simulink model "data_acquisition_file_slider"  (R2019b)
settings: Solver=VariableStepAuto  StartTime=0.0  StopTime=inf  RelTol=1e-3
settings Model: EnablePacing=on  Creator=mandl  LastModifiedBy=mandl

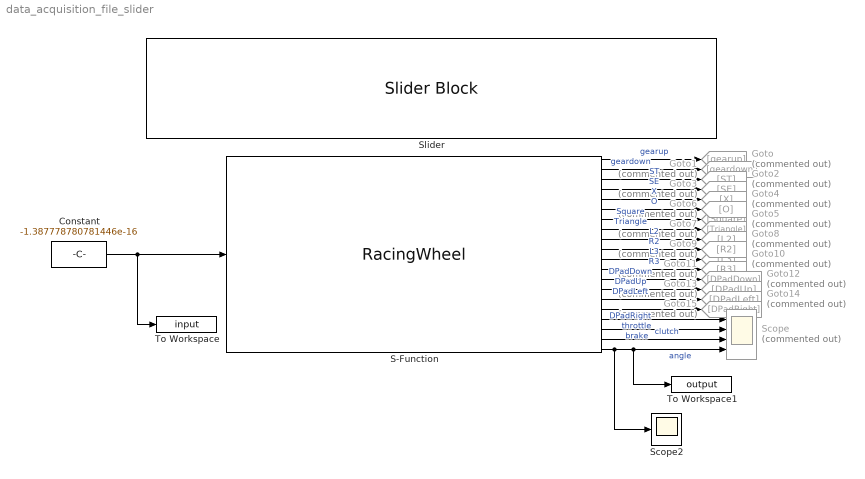
== system data_acquisition_file_slider ==
  Constant : Constant  Value=-1.387778780781446e-16
  Goto : Goto  Commented=on  GotoTag=gearup
  Goto1 : Goto  Commented=on  GotoTag=geardown
  Goto10 : Goto  Commented=on  GotoTag=L3
  Goto11 : Goto  Commented=on  GotoTag=R3
  Goto12 : Goto  Commented=on  GotoTag=DPadDown
  Goto13 : Goto  Commented=on  GotoTag=DPadUp
  Goto14 : Goto  Commented=on  GotoTag=DPadLeft
  Goto15 : Goto  Commented=on  GotoTag=DPadRight
  Goto2 : Goto  Commented=on  GotoTag=ST
  Goto3 : Goto  Commented=on  GotoTag=SE
  Goto4 : Goto  Commented=on  GotoTag=X
  Goto5 : Goto  Commented=on  GotoTag=Square
  Goto6 : Goto  Commented=on  GotoTag=O
  Goto7 : Goto  Commented=on  GotoTag=Triangle
  Goto8 : Goto  Commented=on  GotoTag=L2
  Goto9 : Goto  Commented=on  GotoTag=R2
  S-Function : S-Function  FunctionName=RacingWheel  Parameters=Ts_FF  SFunctionModules=RacingWheel_wrapper  SFunctionDeploymentMode=off  EnableBusSupport=off  mask(Racing Wheel with Force Feedback){Ts_FF=0.01}
      mask prompts: Ts_FF "Constant Force-Feedback Sample Time"
      mask help: Interacts with the windows gaming API from UWP. The force feedback effect is constant over the user defined sampling time below.
      mask init:
      | val = [[.9  0.75 0.75 1 1 .9 .9 1]',[1 1 0.75 0.75 .9 .9 1 .9]'];try , sys = get_param(gcb,'SfunBuilderFcnName');if isempty(sys), sys = get_param(gcb,'FunctionName'); end,catch, sys = get_param(gcb,'FunctionName'); end
      mask Display:
      | plot(val(:,1),val(:,2)),disp(sys),
      | image('icon.png'),
      | port_label('input',1,'FF'),
      | port_label('output',1,'gearup'),
      | port_label('output',2,'geardown'),
      | port_label('output',3,'ST'),
      | port_label('output',4,'SE'),
      | port_label('output',5,'X'),
      | port_label('output',6,'O'),
      | port_label('output',7,'Square'),
      | port_label('output',8,'Triangle'),
      | port_label('output',9,'L2'),
      | port_label('output',10,'R2'),
      | port_label('output',11,'L3'),
      | port_label('output',12,'R3'),
      | port_label('output',13,'DPadDown'),
      | port_label('output',14,'DPadUp'),
      | port_label('output',15,'DPadLeft'),
      | port_label('output',16,'DPadRight'),
      | port_label('output',17,'throttle'),
      | port_label('output',18,'brake'),
      | port_label('output',19,'clutch'),
      | port_label('output',20,'angle')
  Scope : Scope  Commented=on  NumInputPorts=4
  Scope2 : Scope
  Slider : SliderBlock  ScaleMin=-1  ScaleMax=1  TickInterval=0.1
  To Workspace : ToWorkspace  VariableName=input  SaveFormat=Structure With Time  SampleTime=0.01
  To Workspace1 : ToWorkspace  VariableName=output  SaveFormat=Structure With Time  SampleTime=0.01
  wires:
  S-Function/20 -> Scope2/1, To Workspace1/1, Scope/4  "angle"
  S-Function/19 -> Scope/3  "clutch"
  S-Function/18 -> Scope/2  "brake"
  S-Function/17 -> Scope/1  "throttle"
  S-Function/1 -> Goto/1  "gearup"
  S-Function/2 -> Goto1/1  "geardown"
  S-Function/3 -> Goto2/1  "ST"
  S-Function/4 -> Goto3/1  "SE"
  S-Function/5 -> Goto4/1  "X"
  S-Function/6 -> Goto6/1  "O"
  S-Function/7 -> Goto5/1  "Square"
  S-Function/8 -> Goto7/1  "Triangle"
  S-Function/9 -> Goto8/1  "L2"
  S-Function/10 -> Goto9/1  "R2"
  S-Function/11 -> Goto10/1  "L3"
  S-Function/12 -> Goto11/1  "R3"
  S-Function/13 -> Goto12/1  "DPadDown"
  S-Function/14 -> Goto13/1  "DPadUp"
  S-Function/15 -> Goto14/1  "DPadLeft"
  S-Function/16 -> Goto15/1  "DPadRight"
  Constant/1 -> To Workspace/1, S-Function/1
